simulink model "parcialRAMPA"  (R2017b)
settings: Solver=VariableStepAuto  StartTime=0.0  StopTime=10.0  RelTol=1e-3
values from neighbouring files (symbols this model uses):
  Afco = double(A)    [PUNTO1PARCIAL.m]    (also in parcialretro.m)
  Bfco = double(B)    [PUNTO1PARCIAL.m]    (also in parcialretro.m)
  Cfco = double(C)    [PUNTO1PARCIAL.m]    (also in parcialretro.m)
  k1 = eval(Sol.k1)    [PUNTO1PARCIAL.m]    (also in PUNTO1PARCIALLLINTENTO2.m; parcialretro.m)
  k2 = eval(Sol.k2)    [PUNTO1PARCIAL.m]    (also in PUNTO1PARCIALLLINTENTO2.m; parcialretro.m)
  ki = eval(Sol.ki)    [PUNTO1PARCIAL.m]    (also in PUNTO1PARCIALLLINTENTO2.m; Parcial1.m = eval(S.ki); parcialretro.m)
  ki2 = eval(Sol.ki2)    [PUNTO1PARCIAL.m]    (also in Parcial1.m = eval(S.ki2); parcialretro.m)
  L = [PDO(3)-6; PDO(2)-5]    [PUNTO1PARCIAL.m]    (also in parcialretro.m)
libraries: simulink x1
settings Model: Creator=Cx001la  LastModifiedBy=Cx001la

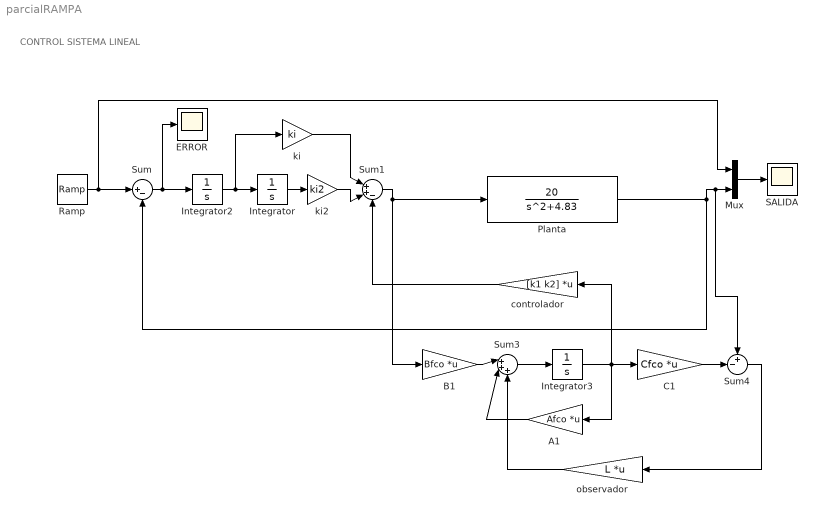
== system parcialRAMPA ==
  note: CONTROL SISTEMA LINEAL
  A1 : Gain  Gain=Afco  Multiplication=Matrix(K*u)
  B1 : Gain  Gain=Bfco  Multiplication=Matrix(K*u)
  C1 : Gain  Gain=Cfco  Multiplication=Matrix(K*u)
  ERROR : Scope
  Integrator : Integrator
  Integrator2 : Integrator
  Integrator3 : Integrator
  Mux : Mux  Inputs=2
  "Planta " : TransferFcn  Numerator=[20]  Denominator=[1 0 4.83]
  Ramp : simulink/Sources/Ramp  slope=1  start=0  X0=0
  SALIDA : Scope
  Sum : Sum  Inputs=|+-
  Sum1 : Sum  Inputs=|++-
  Sum3 : Sum  Inputs=|+++
  Sum4 : Sum  Inputs=+-|
  controlador : Gain  Gain=[k1 k2]  Multiplication=Matrix(K*u)
  ki : Gain  Gain=ki
  ki2 : Gain  Gain=ki2
  "observador " : Gain  Gain=L  Multiplication=Matrix(K*u)
  wires:
  A1/1 -> Sum3/2
  ki/1 -> Sum1/1
  Ramp/1 -> Mux/1, Sum/1
  controlador/1 -> Sum1/3
  Integrator2/1 -> ki/1, Integrator/1
  Sum/1 -> ERROR/1, Integrator2/1
  ki2/1 -> Sum1/2
  Mux/1 -> SALIDA/1
  "observador "/1 -> Sum3/3
  B1/1 -> Sum3/1
  Integrator/1 -> ki2/1
  Sum1/1 -> "Planta "/1, B1/1
  Sum3/1 -> Integrator3/1
  "Planta "/1 -> Sum4/1, Mux/2, Sum/2
  Sum4/1 -> "observador "/1
  C1/1 -> Sum4/2
  Integrator3/1 -> controlador/1, A1/1, C1/1
